simulink model "RealSimTemplate"  (R2024a)
settings: Solver=FixedStepAuto  StartTime=0.0  StopTime=200  FixedStep=0.001  RelTol=1e-3
undefined symbols (not defined in the file or in its folder): RealSimPara
settings Model: Creator=y0n  LastModifiedBy=ys04893
settings SolverCC: AlgebraicLoopSolver=TrustRegion
settings DataIOCC: SaveOutput=off  SignalLogging=off  DSMLogging=off  SaveTime=off  ReturnWorkspaceOutputsName=VehicleOut
settings DebuggingCC: AlgebraicLoopMsg=none  UnconnectedInputMsg=warning  UnconnectedOutputMsg=warning  UnconnectedLineMsg=warning  UnderSpecifiedDimensionMsg=error
settings ModelReferenceCC: EnableRefExpFcnMdlSchedulingChecks=on
settings SFSimCC: CustomCodeUndefinedFunction=UseInterfaceOnly
settings RTWCC: GPUComputeCapability=3.5

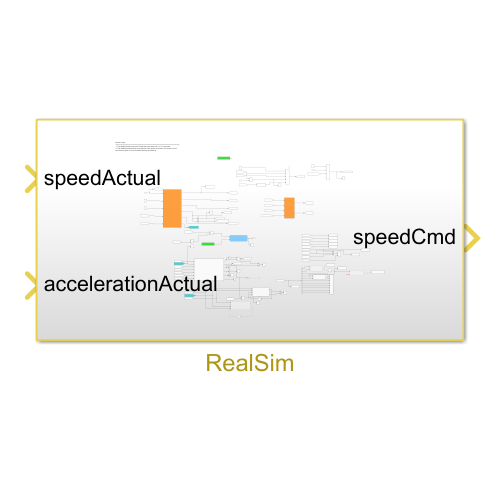
[thumbnail: Simulink's stored preview of the top-level diagram]
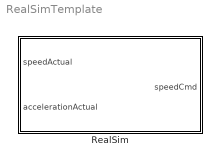
== system RealSimTemplate ==
  RealSim : Subsystem

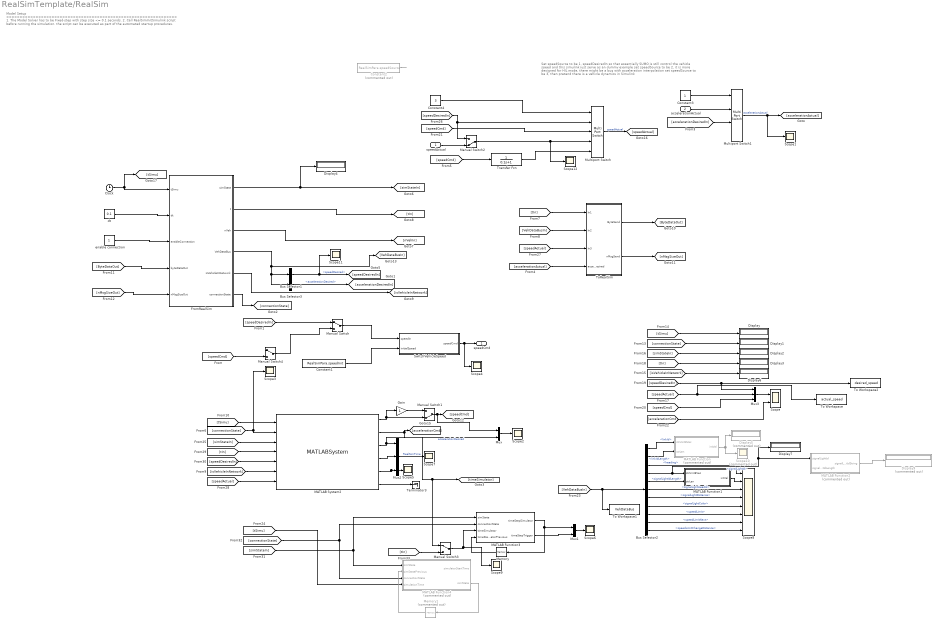
== system RealSimTemplate/RealSim ==
  note: Model Setup
      | ================================================================
      | 1. The Model Solver has to be Fixed-step with step size <= 0.1 seconds.
      | 2. Call RealSimInitSimulink script before running the simulation. the script can be executed as part of the automated startup procedures.
  note: Set speedSource to be 1, speedDesiredIn so that essentially SUMO is still control the vehicle speed and this simulink just serve as an dummy example
      |
      | set speedSource to be 2, it is more designed for HIL mode, there might be a bug with acceleration interpolation
      |
      | set speedSource to be 3, then pretend there is a vehicle dynamics in Simulink
  speedActual : Inport
  accelerationActual : Inport  Port=2
  Bus Selector1 : BusSelector  OutputSignals=speedDesired
  Bus Selector2 : BusSelector  OutputSignals=linkId,linkIdLength,heading,signalLightId,signalLightIdLength,signalLightHeadId,signalLightDistance,signalLightColor,speedLimit,speedLimitNext,speedLimitChangeDistance
  Bus Selector3 : BusSelector  OutputSignals=accelerationDesired
  Clock : Clock
  Constant1 : Constant  Value=RealSimPara.speedInit
  Constant2 : Constant  Commented=on  Value=RealSimPara.speedSource
  Constant3 : Constant
  Constant4 : Constant  Value=3
  Display{,1..4,6..7} (7 alike) : Display
  Display5 : Display  Commented=on
  Display9 : Display  Commented=on
  FromRealSim : Subsystem
  Gain : Gain
  MATLAB Function : MATLAB Function  Commented=on  TreatAsAtomicUnit=on
  MATLAB Function1 : MATLAB Function  TreatAsAtomicUnit=on
  MATLAB Function2 : MATLAB Function  Commented=on  TreatAsAtomicUnit=on  SystemSampleTime=0.001
  MATLAB Function3 : MATLAB Function  TreatAsAtomicUnit=on
  MATLAB Function4 : MATLAB Function  Commented=on  TreatAsAtomicUnit=on
  MATLAB System2 : MATLABSystem  System=RealSimInterpSpeed  initialSpeed=RealSimPara.speedInit  speedLookAheadHorizon=RealSimPara.tLookahead  speedUpperBound=30  smoothWindow=RealSimPara.smoothWindow  SimulateUsing=Interpreted execution
      mask Type: RealSimInterpSpeed
      mask Display:
      | disp('RealSimInterpSpeed');
      | port_label('input',1,'simulationTime');
      | port_label('input',2,'connectionState');
      | port_label('input',3,'simState');
      | port_label('input',4,'timeReceive');
      | port_label('input',5,'speedReceive');
      | port_label('input',6,'isVehicleInNetwork');
      | port_label('input',7,'speedActual');
      | port_label('output',1,'speedLookAhead');
      | port_label('output',2,'accelerationDesired');
      | port_label('output',3,'timeSimulator');
      | port_label('output',4,'timeStepSimulator');
      | port_label('output',5,'timeStepTrigger');
      | port_label('output',6,'RealSimDelay');
  Manual Switch : ManualSwitch
  Manual Switch1 : ManualSwitch  CurrentSetting=0
  Manual Switch2 : ManualSwitch  CurrentSetting=0
  Manual Switch3 : ManualSwitch
  Manual Switch4 : ManualSwitch
  Memory : Memory
  Memory1 : Memory  Commented=on
  Multiport Switch : MultiPortSwitch  Inputs=4  SaturateOnIntegerOverflow=off  InputSameDT=off
  Multiport Switch1 : MultiPortSwitch  SaturateOnIntegerOverflow=off  InputSameDT=off
  Mux : Mux  Inputs=2
  Mux1 : Mux  Inputs=2
  Mux2 : Mux  Inputs=3
  Mux3 : Mux  Inputs=3
  Scope : Scope  NumInputPorts=2
  Scope{1..7,9,11..12} (10 alike) : Scope
  Scope10 : Scope  Commented=on
  Scope8 : Scope  NumInputPorts=8
  SwitchVehicleSpeed : Subsystem
  Terminator3 : Terminator
  To Workspace : ToWorkspace  VariableName=actual_speed  SaveFormat=Timeseries  SampleTime=0.1
  To Workspace1 : ToWorkspace  VariableName=VehDataBus  SaveFormat=Timeseries  SampleTime=-1
  To Workspace2 : ToWorkspace  VariableName=desired_speed  SaveFormat=Timeseries  SampleTime=0.1
  ToRealSim : Subsystem
  Transfer Fcn : TransferFcn  Denominator=[0.1 1]
  dt : Constant  Value=0.1
  enable connection : Constant
  speedCmd : Outport
  wires:
  [tSimu] -> Display/1
  Bus Selector2/5 -> MATLAB Function1/2(strLen)  "<signalLightIdLength>"
  [simStateIn] -> MATLAB System2/3
  [isVehicleInNetwork] -> Display6/1
  [ByteDataOut] -> FromRealSim/4(byteDataOut)
  MATLAB System2/5 -> Scope5/1, Mux2/3
  [VehDataBusIn] -> To Workspace1/1, Bus Selector2/1
  MATLAB System2/1 -> Gain/1, Manual Switch1/2
  [speedCmd] -> Multiport Switch/3
  Mux2/1 -> Scope7/1  "RealSimTime"
  [tSimu] -> MATLAB System2/1
  Gain/1 -> Manual Switch1/1
  Bus Selector1/1 -> Scope11/1, [speedDesiredIn]  "<speedDesired>"
  Bus Selector2/9 -> Scope8/6  "<speedLimit>"
  [speedDesiredIn] -> To Workspace2/1, Mux3/1
  Bus Selector2/4 -> Display7/1, MATLAB Function2/1(signalLightId), MATLAB Function1/1(strUint8Vec)  "<signalLightId>"
  MATLAB System2/3 -> [timeSimulator], Manual Switch3/1, Mux2/1
  dt/1 -> FromRealSim/2(dt)
  Bus Selector2/10 -> Scope8/7  "<speedLimitNext>"
  FromRealSim/4(VehDataBus) -> Bus Selector3/1, Bus Selector1/1, [VehDataBusIn]
  enable connection/1 -> FromRealSim/3(enableConnection)
  MATLAB Function/1(intVal) -> Scope10/1, Display5/1
  [speedDesiredIn] -> MATLAB System2/5
  [nMsgSizeOut] -> FromRealSim/5(nMsgSizeOut)
  Bus Selector2/11 -> Scope8/8  "<speedLimitChangeDistance>"
  [speedDesiredIn] -> Manual Switch2/1, Multiport Switch/2
  [speedActual] -> MATLAB System2/7
  FromRealSim/3(nVeh) -> [nVehIn]
  [speedActual] -> To Workspace/1, Mux3/2
  [connectionState] -> Display1/1
  Clock/1 -> FromRealSim/1(tSimu), [tSimu]
  [tIn] -> Display3/1
  Bus Selector2/7 -> Scope8/4  "<signalLightDistance>"
  MATLAB System2/4 -> Mux2/2
  Bus Selector2/8 -> Scope8/5  "<signalLightColor>"
  Manual Switch2/1 -> Scope12/1, Multiport Switch/4
  [connectionState] -> Scope3/1, MATLAB System2/2
  MATLAB System2/6 -> Terminator3/1
  Bus Selector2/1 -> MATLAB Function/1(strUint8Vec)  "<linkId>"
  [tIn] -> ToRealSim/1(In1)
  MATLAB System2/2 -> [accelerationCmd], Mux/2  "accelerationDesired"
  MATLAB Function2/1(signalLightIdString) -> Display9/1
  Bus Selector2/2 -> MATLAB Function/2(strLen)  "<linkIdLength>"
  [tIn] -> MATLAB System2/4
  [speedCmd] -> Mux3/3
  Constant4/1 -> Multiport Switch/1
  Manual Switch1/1 -> Mux/1, [speedCmd]
  ToRealSim/2(nMsgSend) -> [nMsgSizeOut]
  FromRealSim/1(simState) -> Display4/1, [simStateIn]
  [speedActual] -> ToRealSim/3(In3)
  FromRealSim/2(t) -> [tIn]
  FromRealSim/5(isVehicleInNetwork) -> [isVehicleInNetwork]
  [accelerationCmd] -> Scope/2
  [VehDataBusIn] -> ToRealSim/2(In2)
  Multiport Switch/1 -> [speedActual]  "speedActual"
  Bus Selector2/6 -> Scope8/3  "<signalLightHeadId>"
  [accelerationActual] -> ToRealSim/4(accelerationDesired)
  ToRealSim/1(ByteSend) -> [ByteDataOut]
  MATLAB Function1/1(intVal) -> Scope8/2
  Bus Selector2/3 -> Scope8/1  "<heading>"
  [isVehicleInNetwork] -> MATLAB System2/6
  Mux3/1 -> Scope/1
  [simStateIn] -> Display2/1
  ? -> MATLAB Function2/2(signalLightIdLength)
  Constant2/1 -> ?
  Manual Switch4/1 -> Manual Switch/2
  [speedDesiredIn] -> Manual Switch/1
  Constant1/1 -> SwitchVehicleSpeed/2(initialSpeed)
  SwitchVehicleSpeed/1(speedCmd) -> Scope4/1, speedCmd/1
  Manual Switch/1 -> SwitchVehicleSpeed/1(speedIn)
  Bus Selector3/1 -> [accelerationDesiredIn]  "<accelerationDesired>"
  Constant3/1 -> Multiport Switch1/1
  [accelerationDesiredIn] -> Multiport Switch1/3
  accelerationActual/1 -> Multiport Switch1/2
  Multiport Switch1/1 -> Scope1/1, [accelerationActual]  "accelerationActual"
  FromRealSim/6(connectionState) -> [connectionState]
  Mux/1 -> Scope2/1
  speedActual/1 -> Manual Switch2/2
  [speedCmd] -> Transfer Fcn/1
  Transfer Fcn/1 -> Multiport Switch/5
  [tSimu] -> MATLAB Function4/4(simulationTime)
  [connectionState] -> MATLAB Function4/3(connectionState), MATLAB Function3/2(connectionState)
  [simStateIn] -> MATLAB Function4/1("simState "), MATLAB Function3/1(simState)
  MATLAB Function3/1(timeStepSimulator) -> Mux1/1, Memory/1
  Memory/1 -> MATLAB Function3/4(timeStepSimulatorPrevious)
  Mux1/1 -> Scope6/1
  MATLAB Function3/2(timeStepTrigger) -> Mux1/2
  Memory1/1 -> MATLAB Function4/2(simStatePrevious)
  MATLAB Function4/2(simState) -> Memory1/1
  [tIn] -> Manual Switch3/2
  Manual Switch3/1 -> MATLAB Function3/3(timeSimulator), Scope9/1
  [speedCmd] -> Manual Switch4/2

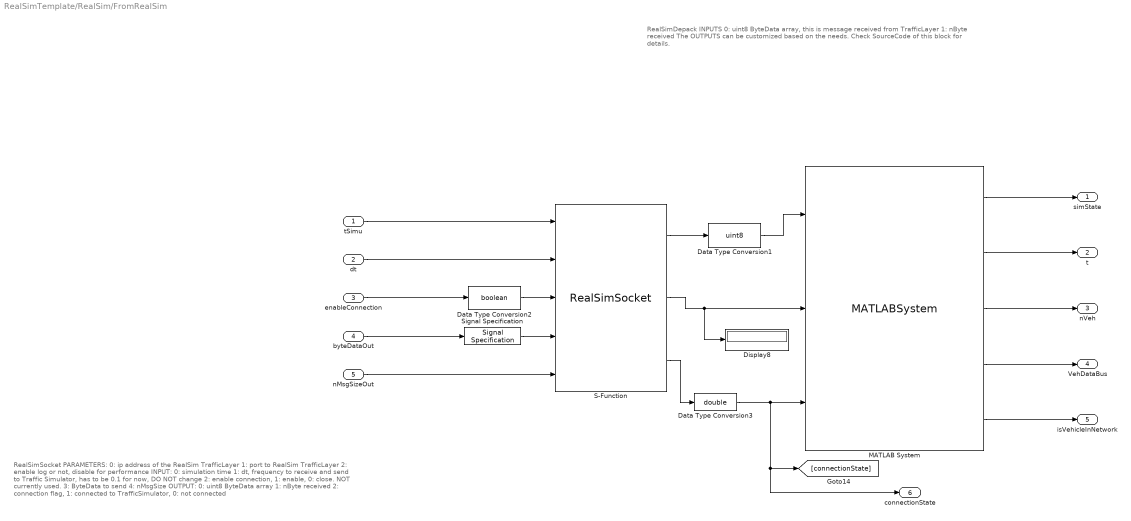
== system RealSimTemplate/RealSim/FromRealSim ==
  note: RealSimSocket
      | PARAMETERS:
      | 0: ip address of the RealSim TrafficLayer
      | 1: port to RealSim TrafficLayer
      | 2: enable log or not, disable for performance
      | INPUT:
      | 0: simulation time
      | 1: dt, frequency to receive and send to Traffic Simulator, has to be 0.1 for now, DO NOT change
      | 2: enable connection, 1: enable, 0: close. NOT currently used.
      | 3: ByteData to send
      | 4: nMsgSize
      |
      | OUTPUT:
      | 0: uint8 ByteData array
      | 1: nByte received
      | 2: connection flag, 1: connected to TrafficSimulator, 0: not connected
  note: RealSimDepack
      | INPUTS
      | 0: uint8 ByteData array, this is message received from TrafficLayer
      | 1: nByte received
      |
      | The OUTPUTS can be customized based on the needs. Check SourceCode of this block for details.
  tSimu : Inport
  dt : Inport  Port=2
  enableConnection : Inport  Port=3
  byteDataOut : Inport  Port=4
  nMsgSizeOut : Inport  Port=5
  Data Type Conversion1 : DataTypeConversion  OutDataTypeStr=uint8  SaturateOnIntegerOverflow=off  RndMeth=Floor
  Data Type Conversion2 : DataTypeConversion  OutDataTypeStr=boolean  SaturateOnIntegerOverflow=off  RndMeth=Floor
  Data Type Conversion3 : DataTypeConversion  OutDataTypeStr=double  SaturateOnIntegerOverflow=off  RndMeth=Floor
  Display8 : Display
  MATLAB System : MATLABSystem  System=RealSimDepack  OutputBusName=VehDataBus  VehicleMessageFieldDefInputVec=VehicleMessageFieldDefInputVec  SimulateUsing=Interpreted execution
      mask Type: RealSimDepack
      mask Display:
      | disp('RealSimDepack');
      | port_label('input',1,'ByteData');
      | port_label('input',2,'nByte');
      | port_label('input',3,'connectionState');
      | port_label('output',1,'simState');
      | port_label('output',2,'t');
      | port_label('output',3,'nVeh');
      | port_label('output',4,'VehDataBus');
      | port_label('output',5,'isVehicleInNetwork');
  S-Function : S-Function  FunctionName=RealSimSocket  Parameters=TrafficLayerIP, TrafficLayerPort, 1  SFunctionDeploymentMode=off  EnableBusSupport=off
  Signal Specification : SignalSpecification  Dimensions=[200 1]
  simState : Outport
  t : Outport  Port=2
  nVeh : Outport  Port=3
  VehDataBus : Outport  Port=4
  isVehicleInNetwork : Outport  Port=5
  connectionState : Outport  Port=6
  wires:
  nMsgSizeOut/1 -> S-Function/5
  S-Function/3 -> Data Type Conversion3/1
  MATLAB System/2 -> t/1
  byteDataOut/1 -> Signal Specification/1
  Data Type Conversion1/1 -> MATLAB System/1
  S-Function/2 -> Display8/1, MATLAB System/2
  Signal Specification/1 -> S-Function/4
  Data Type Conversion2/1 -> S-Function/3
  S-Function/1 -> Data Type Conversion1/1
  MATLAB System/4 -> VehDataBus/1
  MATLAB System/1 -> simState/1
  MATLAB System/3 -> nVeh/1
  MATLAB System/5 -> isVehicleInNetwork/1
  tSimu/1 -> S-Function/1
  dt/1 -> S-Function/2
  enableConnection/1 -> Data Type Conversion2/1
  Data Type Conversion3/1 -> connectionState/1, [connectionState], MATLAB System/3

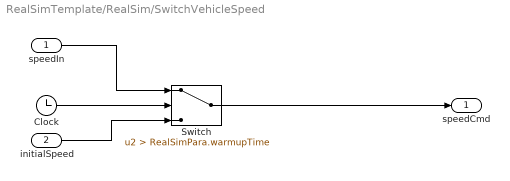
== system RealSimTemplate/RealSim/SwitchVehicleSpeed ==
  speedIn : Inport
  initialSpeed : Inport  Port=2
  Clock : Clock
  Switch : Switch  Criteria=u2 > Threshold  Threshold=RealSimPara.warmupTime  SaturateOnIntegerOverflow=off  InputSameDT=off
  speedCmd : Outport
  wires:
  Switch/1 -> speedCmd/1
  speedIn/1 -> Switch/1
  Clock/1 -> Switch/2
  initialSpeed/1 -> Switch/3

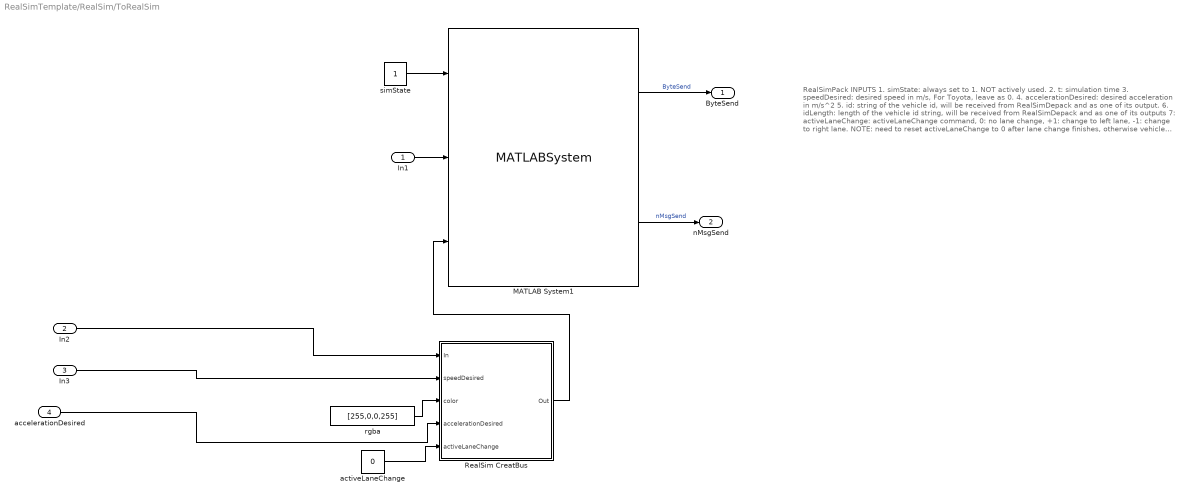
== system RealSimTemplate/RealSim/ToRealSim ==
  note: RealSimPack
      | INPUTS
      | 1. simState: always set to 1. NOT actively used.
      | 2. t: simulation time
      | 3. speedDesired: desired speed in m/s, For Toyota, leave as 0.
      | 4. accelerationDesired: desired acceleration in m/s^2
      | 5. id: string of the vehicle id, will be received from RealSimDepack and as one of its output.
      | 6. idLength: length of the vehicle id string, will be received from RealSimDepack and as one of its outputs
      | 7: activeLaneChange: activeLaneChange command, 0: no lane change, +1: change to left lane, -1: change to right lane. NOTE: need to reset activeLaneChange to 0 after lane change finishes, otherwise vehicle will keep making lane change. Will receive 0 activeLaneChangeFdbk from RealSimDepack when lane change finishes.
      |
      | NOTE 1: Currently, only speedDesired and/or accelerationDesired can be sent to VISSIM/SUMO. The data format receive and send are the same so other mesage fields of the send data are irrelevant and can be set to empty or zero.
      |
      | NOTE 2: if select both speedDesired and accelerationDesired
      | in config.yaml, then only accelerationDesired will be used
      | to control vehicles in TrafficSimulator. if only one of
      | speedDesired and accelerationDesired selected in
      | config.yaml, then the one selected will be used for
      | control, the other input can be leave as 0.
      |
      | NOTE 3: for VISSIM, speedDesired or accelerationDesired will be the control command 0.2 seconds in the future.
      |
      | OUTPUTS
      | 1.ByteData: bytes vector that will be sent to TrafficSimualtor
      | 2.nMsgSize: size of bytes to be sent
  In1 : Inport
  In2 : Inport  Port=2
  In3 : Inport  Port=3
  accelerationDesired : Inport  Port=4
  MATLAB System1 : MATLABSystem  System=RealSimPack  VehicleMessageFieldDefInputVec=VehicleMessageFieldDefInputVec  SimulateUsing=Code generation
      mask Type: RealSimPack
      mask Display:
      | disp('RealSimPack');
      | port_label('input',1,'simState');
      | port_label('input',2,'t');
      | port_label('input',3,'VehDataBus');
      | port_label('output',1,'ByteData');
      | port_label('output',2,'nMsgSize');
  RealSim CreatBus : Subsystem
  activeLaneChange : Constant  Value=0
  rgba : Constant  Value=[255,0,0,255]
  simState : Constant
  ByteSend : Outport
  nMsgSend : Outport  Port=2
  wires:
  rgba/1 -> RealSim CreatBus/3(color)
  MATLAB System1/2 -> nMsgSend/1  "nMsgSend"
  In3/1 -> RealSim CreatBus/2(speedDesired)
  In1/1 -> MATLAB System1/2
  simState/1 -> MATLAB System1/1
  accelerationDesired/1 -> RealSim CreatBus/4(accelerationDesired)
  RealSim CreatBus/1(Out) -> MATLAB System1/3
  activeLaneChange/1 -> RealSim CreatBus/5(activeLaneChange)
  MATLAB System1/1 -> ByteSend/1  "ByteSend"
  In2/1 -> RealSim CreatBus/1(In)

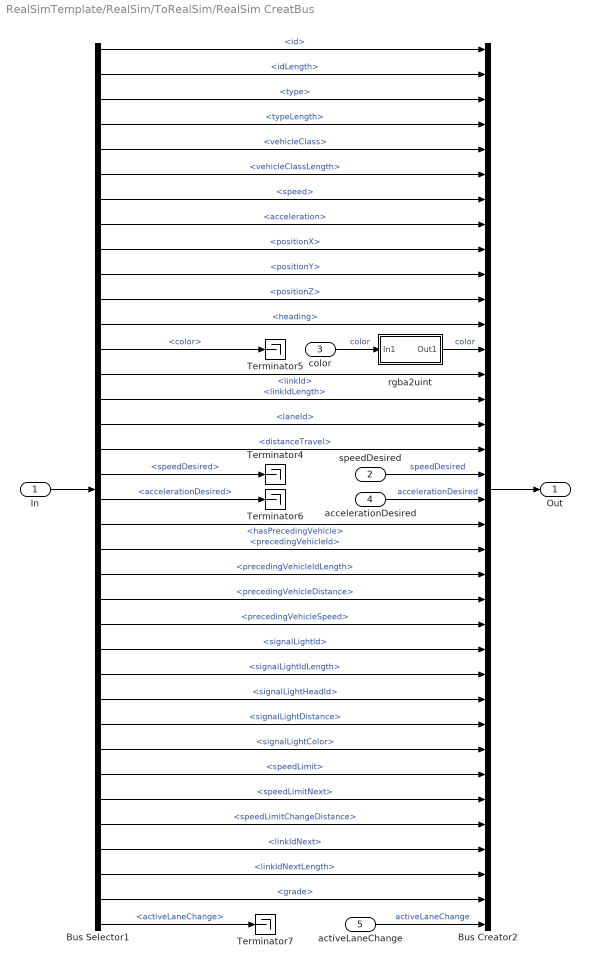
== system RealSimTemplate/RealSim/ToRealSim/RealSim CreatBus ==
  In : Inport
  speedDesired : Inport  Port=2
  color : Inport  Port=3
  accelerationDesired : Inport  Port=4
  activeLaneChange : Inport  Port=5
  Bus Creator2 : BusCreator  Inputs=36  OutDataTypeStr=Bus: VehDataBus
  Bus Selector1 : BusSelector  OutputSignals=id,idLength,type,typeLength,vehicleClass,vehicleClassLength,speed,acceleration,positionX,positionY,positionZ,heading,color,linkId,linkIdLength,laneId,distanceTravel,speedDesired,accelerationDesired,hasPrecedingVehicle,precedingVehicleId,precedingVehicleIdLength,precedingVehicleDistance,precedingVehicleSpeed,signalLightId,signalLightIdLength,signalLightHeadId,signalLightDistance,signalLightColor,speedLimit,speedLimitNext,speedLimitChangeDistance,linkIdNext,linkIdNextLength,grade,activeLaneChange
  Terminator{4..7} (4 alike) : Terminator
  rgba2uint : Subsystem
  Out : Outport
  wires:
  In/1 -> Bus Selector1/1
  Bus Selector1/1 -> Bus Creator2/1  "<id>"
  Bus Selector1/2 -> Bus Creator2/2  "<idLength>"
  Bus Selector1/3 -> Bus Creator2/3  "<type>"
  Bus Selector1/4 -> Bus Creator2/4  "<typeLength>"
  Bus Selector1/5 -> Bus Creator2/5  "<vehicleClass>"
  Bus Selector1/6 -> Bus Creator2/6  "<vehicleClassLength>"
  Bus Selector1/7 -> Bus Creator2/7  "<speed>"
  Bus Selector1/8 -> Bus Creator2/8  "<acceleration>"
  Bus Selector1/9 -> Bus Creator2/9  "<positionX>"
  Bus Selector1/10 -> Bus Creator2/10  "<positionY>"
  Bus Selector1/11 -> Bus Creator2/11  "<positionZ>"
  Bus Selector1/12 -> Bus Creator2/12  "<heading>"
  Bus Selector1/13 -> Terminator5/1  "<color>"
  Bus Selector1/14 -> Bus Creator2/14  "<linkId>"
  Bus Selector1/15 -> Bus Creator2/15  "<linkIdLength>"
  Bus Selector1/16 -> Bus Creator2/16  "<laneId>"
  Bus Selector1/17 -> Bus Creator2/17  "<distanceTravel>"
  Bus Selector1/18 -> Terminator4/1  "<speedDesired>"
  Bus Selector1/19 -> Terminator6/1  "<accelerationDesired>"
  Bus Selector1/20 -> Bus Creator2/20  "<hasPrecedingVehicle>"
  Bus Selector1/21 -> Bus Creator2/21  "<precedingVehicleId>"
  Bus Selector1/22 -> Bus Creator2/22  "<precedingVehicleIdLength>"
  Bus Selector1/23 -> Bus Creator2/23  "<precedingVehicleDistance>"
  Bus Selector1/24 -> Bus Creator2/24  "<precedingVehicleSpeed>"
  Bus Selector1/25 -> Bus Creator2/25  "<signalLightId>"
  Bus Selector1/26 -> Bus Creator2/26  "<signalLightIdLength>"
  Bus Selector1/27 -> Bus Creator2/27  "<signalLightHeadId>"
  Bus Selector1/28 -> Bus Creator2/28  "<signalLightDistance>"
  Bus Selector1/29 -> Bus Creator2/29  "<signalLightColor>"
  Bus Selector1/30 -> Bus Creator2/30  "<speedLimit>"
  Bus Selector1/31 -> Bus Creator2/31  "<speedLimitNext>"
  Bus Selector1/32 -> Bus Creator2/32  "<speedLimitChangeDistance>"
  Bus Selector1/33 -> Bus Creator2/33  "<linkIdNext>"
  Bus Selector1/34 -> Bus Creator2/34  "<linkIdNextLength>"
  Bus Selector1/35 -> Bus Creator2/35  "<grade>"
  Bus Selector1/36 -> Terminator7/1  "<activeLaneChange>"
  activeLaneChange/1 -> Bus Creator2/36  "activeLaneChange"
  speedDesired/1 -> Bus Creator2/18  "speedDesired"
  accelerationDesired/1 -> Bus Creator2/19  "accelerationDesired"
  color/1 -> rgba2uint/1(In1)  "color"
  rgba2uint/1(Out1) -> Bus Creator2/13  "color"
  Bus Creator2/1 -> Out/1

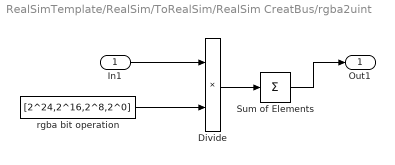
== system RealSimTemplate/RealSim/ToRealSim/RealSim CreatBus/rgba2uint ==
  In1 : Inport
  Divide : Product  Inputs=**
  Sum of Elements : Sum  Inputs=+
  rgba bit operation : Constant  Value=[2^24,2^16,2^8,2^0]
  Out1 : Outport
  wires:
  Divide/1 -> Sum of Elements/1
  In1/1 -> Divide/1
  rgba bit operation/1 -> Divide/2
  Sum of Elements/1 -> Out1/1

== matlab function RealSimTemplate/RealSim/MATLAB Function3 ==
  data: simState input; connectionState input; timeSimulator input; timeStepSimulator output; timeStepSimulatorPrevious input; timeStepTrigger output
function [timeStepSimulator, timeStepTrigger]  = fcn(simState, connectionState, timeSimulator, timeStepSimulatorPrevious)


if simState && abs(connectionState-3) < 1e-5 && (timeSimulator >= timeStepSimulatorPrevious + 0.1 - 1e-5 || abs(timeSimulator) < 1e-5)
    timeStepSimulator = timeSimulator;
    timeStepTrigger = 1;
else
    timeStepSimulator = timeStepSimulatorPrevious;
    timeStepTrigger = 0;
end

== matlab function RealSimTemplate/RealSim/MATLAB Function ==
  data: strUint8Vec input; intVal output double; strLen input
function intVal = strVec2Int(strUint8Vec, strLen)

    strVec = blanks(50);
    for i = 1:strLen
       strVec(i) = strUint8Vec(i); 
    end
    if strLen > 0
        intVal = real(str2double(strVec(1:strLen)));
    else
        intVal = -1;
    end

== matlab function RealSimTemplate/RealSim/MATLAB Function1 ==
  data: strUint8Vec input; intVal output double; strLen input
function intVal = strVec2Int(strUint8Vec, strLen)

    strVec = blanks(50);
    for i = 1:strLen
       strVec(i) = strUint8Vec(i); 
    end
    if strLen > 0
        intVal = real(str2double(strVec(1:strLen)));
    else
        intVal = -1;
    end

== matlab function RealSimTemplate/RealSim/MATLAB Function2 ==
  data: signalLightId input uint8 size=[1 50]; signalLightIdString output string; signalLightIdLength input
function signalLightIdString = fcn(signalLightId, signalLightIdLength)

signalLightIdString = string(char(signalLightId));

== matlab function RealSimTemplate/RealSim/MATLAB Function4 ==
  data: simState input; simulatorStartTime output; simStatePrevious input; connectionState input; simulationTime input; simState output
function [simulatorStartTime, simState] = fcn(simState, simStatePrevious, connectionState, simulationTime)


if abs(simState - 1) < 1e-5 && abs(simStatePrevious) < 1e-5 && abs(connectionState-3) < 1e-5
    % set connectionState and start time
    simulatorStartTime = simulationTime;
else
    simulatorStartTime = 0;
end
